simulink library "constXYZ_TvarSineWave"  (R2018b)
settings: Solver=VariableStepAuto  StartTime=0.0  StopTime=10.0  RelTol=1e-3
undefined symbols (not defined in the file): env
settings Model: Creator=jcreed2  LastModifiedBy=jcreed2

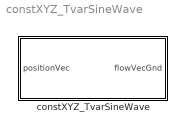
== system constXYZ_TvarSineWave ==
  constXYZ_TvarSineWave : Subsystem

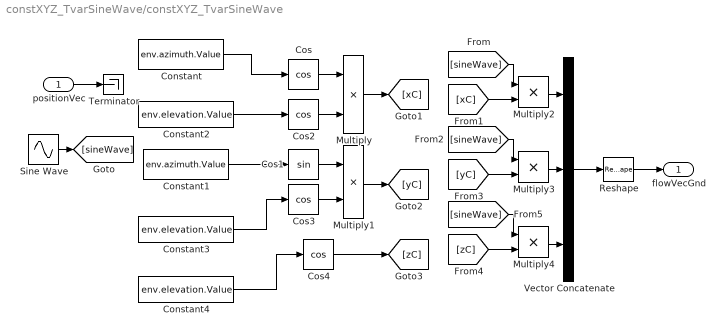
== system constXYZ_TvarSineWave/constXYZ_TvarSineWave ==
  "positionVec " : Inport
  Constant : Constant  Value=env.azimuth.Value
  Constant1 : Constant  Value=env.azimuth.Value
  Constant2 : Constant  Value=env.elevation.Value
  Constant3 : Constant  Value=env.elevation.Value
  Constant4 : Constant  Value=env.elevation.Value
  Cos{,2..4} (4 alike) : Trigonometry  Operator=cos
  Cos1 : Trigonometry
  Multiply{,1..4} (5 alike) : Product
  Reshape : Reshape  OutputDimensionality=Column vector (2-D)
  Sine Wave : Sin  Amplitude=env.amplitude.Value  Bias=env.waveBias.Value  Frequency=env.frequency.Value  Phase=env.phase.Value  SampleTime=0
  Terminator : Terminator
  Vector Concatenate : Concatenate  NumInputs=3
  flowVecGnd : Outport
  wires:
  Reshape/1 -> flowVecGnd/1
  "positionVec "/1 -> Terminator/1
  Vector Concatenate/1 -> Reshape/1
  Multiply/1 -> [xC]
  Cos/1 -> Multiply/1
  Constant/1 -> Cos/1
  Cos1/1 -> Multiply1/1
  Constant1/1 -> Cos1/1
  Sine Wave/1 -> [sineWave]
  Multiply1/1 -> [yC]
  Cos2/1 -> Multiply/2
  Constant2/1 -> Cos2/1
  Cos3/1 -> Multiply1/2
  Constant3/1 -> Cos3/1
  Constant4/1 -> Cos4/1
  Cos4/1 -> [zC]
  Multiply2/1 -> Vector Concatenate/1
  [sineWave] -> Multiply2/1
  [xC] -> Multiply2/2
  [sineWave] -> Multiply3/1
  [yC] -> Multiply3/2
  Multiply3/1 -> Vector Concatenate/2
  Multiply4/1 -> Vector Concatenate/3
  [zC] -> Multiply4/2
  [sineWave] -> Multiply4/1
